simulink model "FlutterSuppressionSystem"  (R2022b)
settings: Solver=ode45  StartTime=0  StopTime=15.01  FixedStep=ts  MaxStep=0.003  RelTol=1e-3  EnableMultiTasking=on
model workspace (MAT data in the model file):
  ts = 0.001
undefined symbols (not defined in the file or in its folder): Hecate_Alt, Hecate_Mach, X, Y, Z
libraries: nesl_utility x14, sm_lib x11, simulink x3, aerolibprivatev1p5 x1, aerolibasang x1
settings Model: Creator=The MathWorks, Inc.  LastModifiedBy=fedformi_new
settings SolverCC: ConcurrentTasks=on  AlgebraicLoopSolver=TrustRegion  PositivePriorityOrder=on  AutoInsertRateTranBlk=on  InsertRTBMode=Never (minimum delay)
settings DataIOCC: SaveFormat=Array  TimeSaveName=tOut  OutputSaveName=yOut  SignalLoggingName=sigsOut
settings OptimizationCC: BlockReduction=off  OptimizeBlockIOStorage=off  BufferReuse=off  GlobalBufferReuse=off  ExpressionFolding=off  ExpressionDepthLimit=2147483647  LocalBlockOutputs=off  InitFltsAndDblsToZero=on  OptimizeDataStoreBuffers=off  BusAssignmentInplaceUpdate=off
settings DebuggingCC: AlgebraicLoopMsg=none  SaveWithParameterizedLinksMsg=none  UnderspecifiedInitializationDetection=Classic  MergeDetectMultiDrivingBlocksExec=none  SignalResolutionControl=TryResolveAllWithWarning  FcnCallInpInsideContextMsg=warning  StateNameClashWarn=warning  SFUnexpectedBacktrackingDiag=warning  SFNoUnconditionalDefaultTransitionDiag=warning  SFExecutionAtInitializationDiag=none  SFMachineParentedDataDiag=warning  ArithmeticOperatorsInVariantConditions=warning
settings ModelReferenceCC: EnableRefExpFcnMdlSchedulingChecks=on  PropagateSignalLabelsOutOfModel=off
settings SFSimCC: SimUseLocalCustomCode=off  SimParseCustomCode=off  CustomCodeUndefinedFunction=UseInterfaceOnly
settings RTWCC: RTWUseLocalCustomCode=off  BuildConfiguration=Faster Runs  DLArmComputeVersion=19.05
settings CodeAppCC: StateflowObjectComments=on
settings ConfigComp: CovMetricSettings=dw  CovSaveCumulativeToWorkspaceVar=on  CovSaveSingleToWorkspaceVar=on  CovExternalEMLEnable=off  CovSFcnEnable=off
settings SimscapeCC: SimscapeNormalizeSystem=off
settings ConfigurationSet: Description=SimMechanics 2G
settings ExplorerConfigSet: SimMechanicsOpenEditorOnUpdate=off

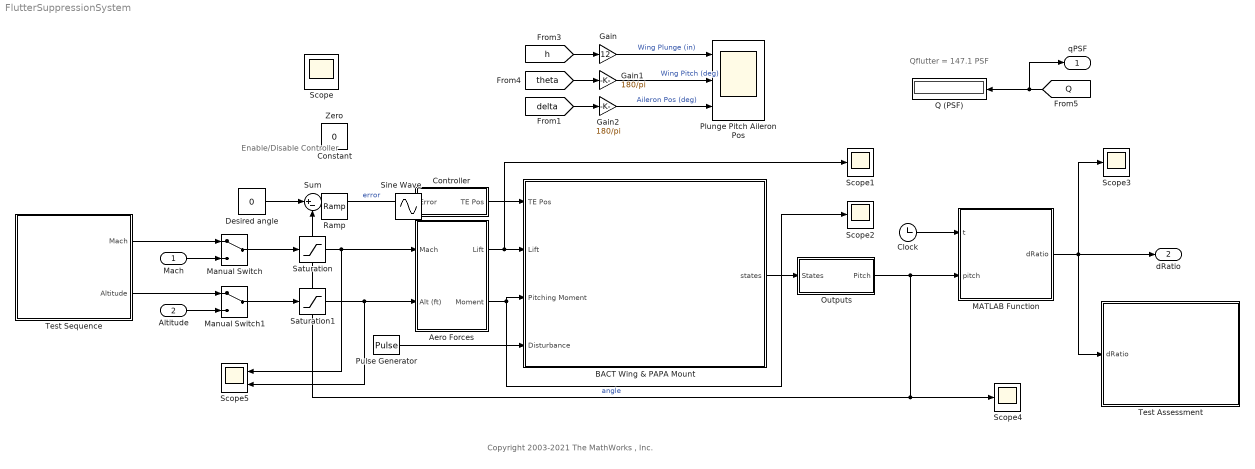
== system FlutterSuppressionSystem ==
  note: Copyright 2003-2021 The MathWorks , Inc.
  note: Enable/Disable Controller
  note: Qflutter = 147.1 PSF
  Mach : Inport
  Altitude : Inport  Port=2
  Aero Forces : Subsystem
  BACT Wing & PAPA Mount : Subsystem  mask{m=6.08, iyy=2.8, Kp=2686.0, zetaP=.0014*2*6.08*21.01, Kt=3000.0, zetaT=.001*2*2.8*32.71, xcg=-.175/100*1.33}
      mask prompts: m "Mass (slug)"; iyy "Inertia (slug*ft^2)"; Kp "PAPA Plunge Stiffness (lb/ft)"; zetaP "PAPA Plunge Damping"; Kt "PAPA Pitch Stiffness (ft-lb)"; zetaT "PAPA Pitch Damping"; xcg "CG Distance from Elastic Axis (+aft)"
      mask Display:
      | image('BACTwing.jpg')
      | port_label('input',1,'TE Position (deg)')
      | port_label('input',2,'Lift')
      | port_label('input',3,'Pitching Moment')
      | port_label('input',4,'Initial Disturbance')
      | port_label('output',1,'States')
  Clock : Clock
  Controller : Subsystem
  Desired angle : Constant  Value=0
  Gain : Gain  Gain=12
  Gain1 : Gain  Gain=180/pi
  Gain2 : Gain  Gain=180/pi
  MATLAB Function : MATLAB Function  TreatAsAtomicUnit=on
  Manual Switch : ManualSwitch
  Manual Switch1 : ManualSwitch
  Outputs : Subsystem
  Plunge Pitch Aileron Pos : Scope  NumInputPorts=3
  Pulse Generator : DiscretePulseGenerator  PulseType=Time based  Amplitude=-10+3*rand  Period=30  PulseWidth=0.05  PhaseDelay=2+3*rand
  Q (PSF) : Display
  Saturation : Saturate  UpperLimit=1  LowerLimit=0.1
  Saturation1 : Saturate  UpperLimit=51000  LowerLimit=1000
  Scope{,1..4} (5 alike) : Scope
  Scope5 : Scope  NumInputPorts=2
  Sum : Sum  Inputs=|+-
  Test Assessment : Test Sequence  TreatAsAtomicUnit=on
  Test Sequence : Test Sequence  TreatAsAtomicUnit=on
  qPSF : Outport  VectorParamsAs1DForOutWhenUnconnected=off
  dRatio : Outport  Port=2
  Constant : Constant  IOType=siggen  Value=-1
  Ramp : simulink/Sources/Ramp  IOType=siggen  slope=1  start=0  InitialOutput=0
  Sine Wave : Sin  IOType=siggen  Amplitude=10  Frequency=5  Phase=pi/2  SampleTime=0
  Zero : Constant  IOType=siggen  Value=0
  wires:
  Manual Switch1/1 -> Saturation1/1
  Manual Switch/1 -> Saturation/1
  BACT Wing & PAPA Mount/1(states) -> Outputs/1(States)
  [Q] -> Q (PSF)/1, qPSF/1
  [h] -> Gain/1
  [theta] -> Gain1/1
  Gain/1 -> Plunge Pitch Aileron Pos/1  "Wing Plunge (in)"
  Gain1/1 -> Plunge Pitch Aileron Pos/2  "Wing Pitch (deg)"
  Sum/1 -> Controller/1(Error)  "error"
  Outputs/1(Pitch) -> MATLAB Function/2(pitch), Sum/2, Scope4/1  "angle"
  Controller/1(TE Pos) -> BACT Wing & PAPA Mount/1(TE Pos)
  [delta] -> Gain2/1
  Gain2/1 -> Plunge Pitch Aileron Pos/3  "Aileron Pos (deg)"
  Desired angle/1 -> Sum/1
  Pulse Generator/1 -> BACT Wing & PAPA Mount/4(Disturbance)
  Aero Forces/1(Lift) -> Scope1/1, BACT Wing & PAPA Mount/2(Lift)
  Aero Forces/2(Moment) -> BACT Wing & PAPA Mount/3(Pitching Moment), Scope2/1
  Clock/1 -> MATLAB Function/1(t)
  Test Sequence/1(Mach) -> Manual Switch/1
  Mach/1 -> Manual Switch/2
  Test Sequence/2(Altitude) -> Manual Switch1/1
  Altitude/1 -> Manual Switch1/2
  MATLAB Function/1(dRatio) -> Scope3/1, dRatio/1, Test Assessment/1(dRatio)
  Saturation/1 -> Scope5/1, Aero Forces/1(Mach)
  Saturation1/1 -> Scope5/2, Aero Forces/2(Alt (ft))

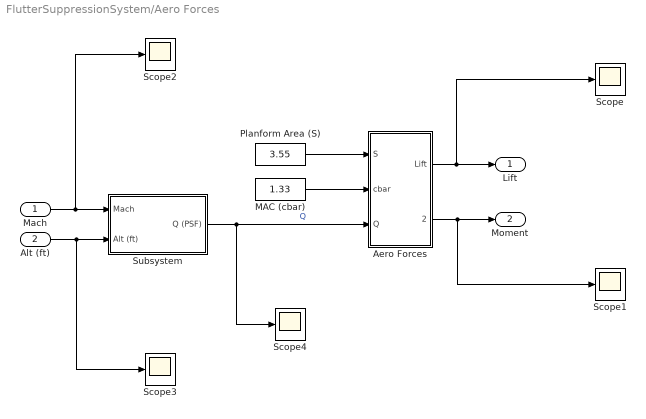
== system FlutterSuppressionSystem/Aero Forces ==
  Mach : Inport
  Alt (ft) : Inport  Port=2
  Aero Forces : Subsystem
  MAC (cbar) : Constant  Value=1.33
  Planform Area (S) : Constant  Value=3.55
  Scope{,1..4} (5 alike) : Scope
  Subsystem : Subsystem
  Lift : Outport  VectorParamsAs1DForOutWhenUnconnected=off
  Moment : Outport  Port=2  VectorParamsAs1DForOutWhenUnconnected=off
  wires:
  MAC (cbar)/1 -> Aero Forces/2(cbar)
  Planform Area (S)/1 -> Aero Forces/1(S)
  Subsystem/1(Q (PSF)) -> Scope4/1, Aero Forces/3(Q)  "Q"
  Aero Forces/1(Lift) -> Scope/1, Lift/1
  Mach/1 -> Scope2/1, Subsystem/1(Mach)
  Aero Forces/2(Moment) -> Scope1/1, Moment/1
  Alt (ft)/1 -> Scope3/1, Subsystem/2(Alt (ft))

== system FlutterSuppressionSystem/BACT Wing & PAPA Mount ==
  TE Pos : Inport
  Lift : Inport  Port=2
  Pitching Moment : Inport  Port=3
  Disturbance : Inport  Port=4
  Bus Creator : BusCreator  Inputs=6
  Mux1 : Mux  Inputs=6
  Sum : Sum  Inputs=++|
  Trailing Edge : Subsystem
  Wing/PAPA Mount : Subsystem
  states : Outport  VectorParamsAs1DForOutWhenUnconnected=off
  wires:
  Bus Creator/1 -> states/1
  Mux1/1 -> Wing/PAPA Mount/1(Aerodynamic Forces)
  Lift/1 -> Mux1/5
  Pitching Moment/1 -> Sum/2
  Sum/1 -> Mux1/3
  Wing/PAPA Mount/1(h) -> Bus Creator/1
  Wing/PAPA Mount/2(hDot) -> Bus Creator/2
  Wing/PAPA Mount/3(theta) -> Bus Creator/3
  Wing/PAPA Mount/4(thetaDot) -> Bus Creator/4
  Trailing Edge/1(delta) -> Bus Creator/5
  Trailing Edge/2(deltaDot) -> Bus Creator/6
  TE Pos/1 -> Trailing Edge/1(TE Pos)
  Disturbance/1 -> Sum/1
  connections:
  Trailing Edge/LConn1 -- Wing/PAPA Mount/RConn1

== system FlutterSuppressionSystem/Controller ==
  Error : Inport
  Constant : Constant
  Enabled Subsystem : Subsystem  TreatAsAtomicUnit=on
  Physical Constraints : Subsystem  mask(Physical Constraint Block){satLimit=15, rateLimit=15/.05*2}
      mask prompts: satLimit "Maximum Deflection (+/- n deg)"; rateLimit "Maximum Deflection Rate (+/- n deg/sec)"
      mask help:
      | In place of an actual actuator model, this block enforces the following constraints:
      | 1 - Maximum/Minimum deflection angle in degrees.
      | 2 - Maximum deflection rate in degrees/sec.
  on/off : Gain  Gain=1.0
  TE Pos : Outport  VectorParamsAs1DForOutWhenUnconnected=off
  wires:
  Enabled Subsystem/1(teCMD) -> Physical Constraints/1(command)  "TE command"
  Error/1 -> Enabled Subsystem/1(error)
  Physical Constraints/1(actual) -> TE Pos/1
  on/off/1 -> Enabled Subsystem/Enable
  Constant/1 -> on/off/1

== system FlutterSuppressionSystem/Outputs ==
  States : Inport
  Bus Selector : BusSelector  OutputSignals=h,hDot,theta,thetaDot,delta,deltaDot
  Memory : Memory
  Pitch : Outport  VectorParamsAs1DForOutWhenUnconnected=off
  tag scope: delta=global, deltaDot=global, h=global, hDot=global, theta=global, thetaDot=global
  wires:
  Bus Selector/1 -> [h]  "<h>"
  Bus Selector/2 -> [hDot]  "<hDot>"
  Bus Selector/3 -> [theta], Memory/1  "<theta>"
  Bus Selector/4 -> [thetaDot]  "<thetaDot>"
  Bus Selector/5 -> [delta]  "<delta>"
  Bus Selector/6 -> [deltaDot]  "<deltaDot>"
  States/1 -> Bus Selector/1
  Memory/1 -> Pitch/1

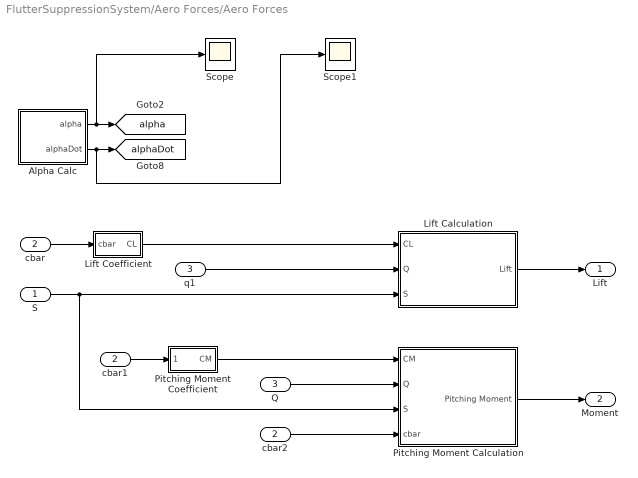
== system FlutterSuppressionSystem/Aero Forces/Aero Forces ==
  S : Inport
  cbar : Inport  Port=2
  Q : Inport  Port=3
  Alpha Calc : Subsystem
  Lift Coefficient : Subsystem
  Lift Calculation : Subsystem
  Pitching Moment Coefficient : Subsystem
  Pitching Moment Calculation : Subsystem
  Scope : Scope
  Scope1 : Scope
  cbar1 : InportShadow  Port=2
  cbar2 : InportShadow  Port=2
  q1 : InportShadow  Port=3
  Lift : Outport  VectorParamsAs1DForOutWhenUnconnected=off
  Moment : Outport  Port=2  VectorParamsAs1DForOutWhenUnconnected=off
  tag scope: alpha=global, alphaDot=global
  wires:
  Lift Coefficient/1(CL) -> Lift Calculation/1(CL)
  q1/1 -> Lift Calculation/2(Q)
  Pitching Moment Coefficient/1(CM) -> Pitching Moment Calculation/1(CM)
  S/1 -> Pitching Moment Calculation/3(S), Lift Calculation/3(S)
  Lift Calculation/1(Lift) -> Lift/1
  Pitching Moment Calculation/1(Pitching Moment) -> Moment/1
  Q/1 -> Pitching Moment Calculation/2(Q)
  cbar/1 -> Lift Coefficient/1(cbar)
  cbar1/1 -> Pitching Moment Coefficient/1(cbar)
  cbar2/1 -> Pitching Moment Calculation/4(cbar)
  Alpha Calc/2(alphaDot) -> Scope1/1, [alphaDot]
  Alpha Calc/1(alpha) -> Scope/1, [alpha]

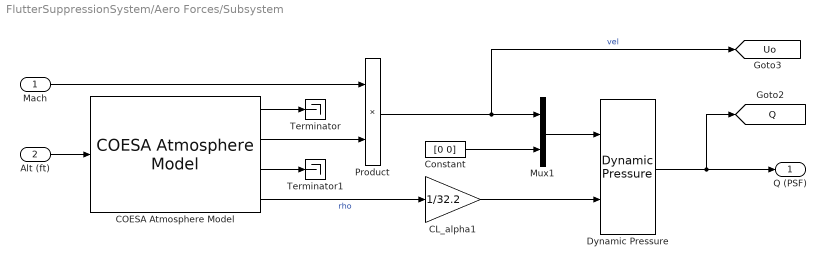
== system FlutterSuppressionSystem/Aero Forces/Subsystem ==
  Mach : Inport
  Alt (ft) : Inport  Port=2
  CL_alpha1 : Gain  Gain=1/32.2  SaturateOnIntegerOverflow=on  OutDataTypeStr=Inherit: Same as input  ParamDataTypeStr=Inherit: Same as input
  COESA Atmosphere Model : aerolibprivatev1p5/COESA Atmosphere Model  units=English
  Constant : Constant  Value=[0 0]
  Dynamic Pressure : aerolibasang/Dynamic Pressure
  Mux1 : Mux  Inputs=2
  Product : Product  SaturateOnIntegerOverflow=on  OutDataTypeStr=Inherit: Same as first input
  Terminator : Terminator
  Terminator1 : Terminator
  Q (PSF) : Outport  VectorParamsAs1DForOutWhenUnconnected=off
  tag scope: Q=global, Uo=global
  wires:
  COESA Atmosphere Model/1 -> Terminator/1
  COESA Atmosphere Model/3 -> Terminator1/1
  COESA Atmosphere Model/2 -> Product/2
  COESA Atmosphere Model/4 -> CL_alpha1/1  "rho"
  Product/1 -> [Uo], Mux1/1  "vel"
  Alt (ft)/1 -> COESA Atmosphere Model/1
  Constant/1 -> Mux1/2
  Mach/1 -> Product/1
  Mux1/1 -> Dynamic Pressure/1
  CL_alpha1/1 -> Dynamic Pressure/2
  Dynamic Pressure/1 -> [Q], Q (PSF)/1

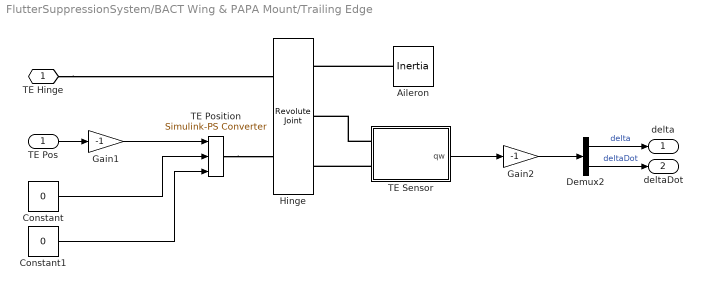
== system FlutterSuppressionSystem/BACT Wing & PAPA Mount/Trailing Edge ==
  TE Pos : Inport
  Aileron : sm_lib/Body Elements/Inertia  InertiaType=Custom  Mass=(1e-9)*14.5939  MassUnits=kg  CenterOfMass=[-8 0 0]  CenterOfMassUnits=in  MomentsOfInertia=([1 1 1]*1e-9)*1.35581795  MomentsOfInertiaUnits=kg*m^2  ProductsOfInertia=[0 0 0]  ProductsOfInertiaUnits=kg*m^2  GraphicType=Marker  MarkerShape=Inertia  MarkerSize=20  GraphicVisPropType=SimpleVisualProperties  GraphicDiffuseColor=[0.5 0.5 0.5]  GraphicSpecularColor=[0.5 0.5 0.5 1.0]  GraphicAmbientColor=[0.15 0.15 0.15 1.0]  GraphicEmissiveColor=[0.0 0.0 0.0 1.0]  GraphicShininess=75  GraphicOpacity=1.0
  Constant : Constant  Value=0
  Constant1 : Constant  Value=0
  Demux2 : Demux  Outputs=2
  Gain1 : Gain  Gain=-1
  Gain2 : Gain  Gain=-1
  Hinge : sm_lib/Joints/Revolute Joint  JointMode=Normal  SenseConstraintForce=off  SenseConstraintForceX=off  SenseConstraintForceY=off  SenseConstraintForceZ=off  SenseConstraintTorque=off  SenseConstraintTorqueX=off  SenseConstraintTorqueY=off  SenseConstraintTorqueZ=off  SenseTotalForce=off  SenseTotalForceX=off  SenseTotalForceY=off  SenseTotalForceZ=off  SenseTotalTorque=off  SenseTotalTorqueX=off  SenseTotalTorqueY=off  SenseTotalTorqueZ=off  CompositeWrenchDir=FollowerOnBase  CompositeWrenchFrame=BaseFrame  EquilibriumPosition=0  EquilibriumPositionUnits=deg  SpringStiffness=0  SpringStiffnessUnits=N*m/deg  DampingCoefficient=0  DampingCoefficientUnits=N*m/(deg/s)  TorqueActuationMode=ComputedTorque  MotionActuationMode=InputMotion  SensePosition=on  SenseVelocity=on  SenseAcceleration=off  SenseTorqueForce=off  SenseLowerLimitTorqueForce=off  SenseUpperLimitTorqueForce=off  LowerLimitSpecify=off  LowerLimitBound=-90  LowerLimitBoundUnits=deg  LowerLimitStiffness=1e4  LowerLimitStiffnessUnits=N*m/deg  LowerLimitDamping=10  LowerLimitDampingUnits=N*m/(deg/s)  LowerLimitTransitionRegionWidth=0.1  LowerLimitTransitionRegionWidthUnits=deg  UpperLimitSpecify=off  UpperLimitBound=90  UpperLimitBoundUnits=deg  UpperLimitStiffness=1e4  UpperLimitStiffnessUnits=N*m/deg  UpperLimitDamping=10  UpperLimitDampingUnits=N*m/(deg/s)  UpperLimitTransitionRegionWidth=0.1  UpperLimitTransitionRegionWidthUnits=deg  PositionTargetSpecify=off  PositionTargetPriority=High  PositionTargetValue=0  PositionTargetValueUnits=deg  VelocityTargetSpecify=off  VelocityTargetPriority=High  VelocityTargetValue=0  VelocityTargetValueUnits=deg/s
  TE Position : nesl_utility/Simulink-PS Converter  PhysicalDomain=network_engine_domain  SubClassName=ps_input  LeftPortType=input  RightPortType=output  PseudoPeriodic=off  Frequencies=[]  NoiseDistribution=none  NoiseParameters=[]  Unit=deg  AffineConversion=off  FilteringAndDerivatives=provide  SimscapeFilterOrder=2  InputFilterTimeConstant=0.001  UdotUserProvided=2
  TE Sensor : Subsystem
  TE Hinge : PMIOPort  Side=Left
  delta : Outport  VectorParamsAs1DForOutWhenUnconnected=off
  deltaDot : Outport  Port=2  VectorParamsAs1DForOutWhenUnconnected=off
  wires:
  Gain2/1 -> Demux2/1
  TE Pos/1 -> Gain1/1
  Demux2/1 -> delta/1  "delta"
  Demux2/2 -> deltaDot/1  "deltaDot"
  Gain1/1 -> TE Position/1
  TE Sensor/1(qw) -> Gain2/1
  Constant/1 -> TE Position/2
  Constant1/1 -> TE Position/3
  connections:
  TE Position/RConn1 -- Hinge/LConn2
  Aileron/RConn1 -- Hinge/RConn1
  TE Sensor/LConn1 -- Hinge/RConn2
  TE Sensor/LConn2 -- Hinge/RConn3
  TE Hinge/RConn1 -- Hinge/LConn1

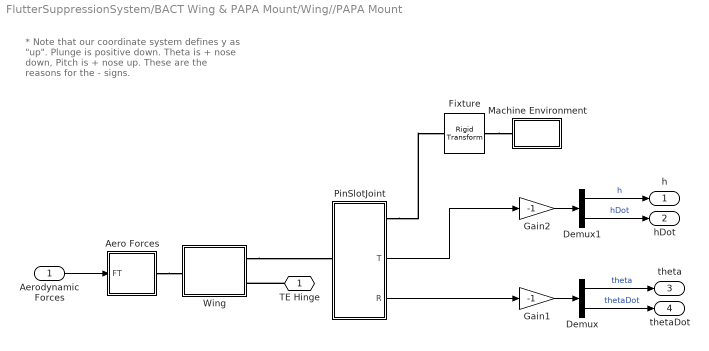
== system FlutterSuppressionSystem/BACT Wing & PAPA Mount/Wing//PAPA Mount ==
  note: * Note that our coordinate system
      | defines y as "up".  Plunge is positive down.
      | Theta is + nose down, Pitch is + nose up.
      | These are the reasons for the - signs.
  Aerodynamic Forces : Inport
  Aero Forces : Subsystem
  Demux : Demux  Outputs=2
  Demux1 : Demux  Outputs=2
  Fixture : sm_lib/Frames and Transforms/Rigid Transform  TranslationMethod=Cartesian  TranslationStandardOffset=0  TranslationLengthUnit=in  TranslationStandardAxis=+Z  TranslationCartesianOffset=[4 0 0]  TranslationROffset=0  TranslationROffsetUnits=m  TranslationZOffset=0  TranslationZOffsetUnits=m  TranslationThetaOffset=0  TranslationThetaOffsetUnits=deg  RotationMethod=None  RotationAngleUnits=deg  RotationStandardAxis=+Z  RotationAngle=0.0  RotationArbitraryAxis=[0 0 1]  FollAlignAxisA=+X  BaseAlignAxisA=+Y  FollAlignAxisB=+Y  BaseAlignAxisB=+Z  RotationSequenceAxes=FollowerAxes  RotationSequence=XYX  RotationSequenceAngles=[0 0 0]  RotationSequenceAnglesUnits=deg  RotationMatrix=[1 0 0; 0 1 0; 0 0 1]  Quaternion=[1 0 0 0]
  Gain1 : Gain  Gain=-1
  Gain2 : Gain  Gain=-1
  Machine Environment : Subsystem
  PinSlotJoint : Subsystem
      settings: PortSchema="{\"entries\":[{\"content\":{\"sides\":[{\"content\":{\"connectorIds\":[\"LConn1\",\"Out1\",\"Out2\"]},\"type\":\"ConnectorPlacement.EquallySpacedRectSide\",\"uuid\":\"cdb19b1c-c324-4790-bce0-6ea35c5c238f\"},{\"content\":{\"connectorIds\":[\"RConn1\"],\"side\":\"RIGHT\"},\"type\":\"ConnectorPlacement.EquallySpacedRectSide\",\"uuid\":\"403fc385-ba39-4b7a-a6e6-6154bbf75764\"},{\"content\":{\"connectorIds\":[],\"side\":\"TOP\"},\"type\":\"ConnectorPlacement.EquallySpacedRectSide\",\"uuid\":\"fec16613-0661-475b-a896-54521c2e84d5\"}]},\"type\":\"ConnectorPlacement.EquallySpacedConnector\",\"uuid\":\"b146dd63-fc25-4a76-acd3-1d9d241f42f8\"}],\"packageUris\":[\"http://schema.mathworks.com/mf0/Connector/19700101\"],\"version\":\"1.0\"}"
  Wing : Subsystem
  TE Hinge : PMIOPort  Side=Right
  h : Outport  VectorParamsAs1DForOutWhenUnconnected=off
  hDot : Outport  Port=2  VectorParamsAs1DForOutWhenUnconnected=off
  theta : Outport  Port=3  VectorParamsAs1DForOutWhenUnconnected=off
  thetaDot : Outport  Port=4  VectorParamsAs1DForOutWhenUnconnected=off
  wires:
  PinSlotJoint/2(R) -> Gain1/1
  PinSlotJoint/1(T) -> Gain2/1
  Demux1/1 -> h/1  "h"
  Demux1/2 -> hDot/1  "hDot"
  Demux/1 -> theta/1  "theta"
  Demux/2 -> thetaDot/1  "thetaDot"
  Gain1/1 -> Demux/1
  Gain2/1 -> Demux1/1
  Aerodynamic Forces/1 -> Aero Forces/1(FT)
  connections:
  Fixture/LConn1 -- Machine Environment/LConn1
  PinSlotJoint/LConn1 -- Fixture/RConn1
  Wing/RConn1 -- PinSlotJoint/RConn1
  Aero Forces/RConn1 -- Wing/LConn1
  TE Hinge/RConn1 -- Wing/RConn2

== system FlutterSuppressionSystem/Controller/Enabled Subsystem ==
  error : Inport
  Enable : EnablePort  StatesWhenEnabling=reset
  Controller : TransferFcn  Numerator=[-10393.7989539677 -80183.6874752132 -565082.359817244]  Denominator=[1 100 0]
  teCMD : Outport  VectorParamsAs1DForOutWhenUnconnected=off
  wires:
  error/1 -> Controller/1
  Controller/1 -> teCMD/1

== system FlutterSuppressionSystem/Controller/Physical Constraints ==
  command : Inport
  Rate Limiter : RateLimiter  RisingSlewLimit=rateLimit  FallingSlewLimit=-rateLimit  SampleTimeMode=inherited
  Saturation : Saturate  UpperLimit=satLimit  LowerLimit=-satLimit
  actual : Outport  VectorParamsAs1DForOutWhenUnconnected=off
  wires:
  Saturation/1 -> Rate Limiter/1
  Rate Limiter/1 -> actual/1
  command/1 -> Saturation/1

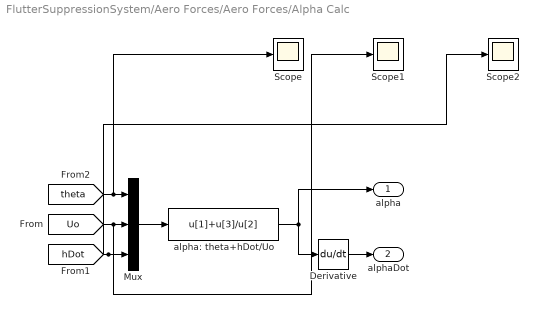
== system FlutterSuppressionSystem/Aero Forces/Aero Forces/Alpha Calc ==
  Derivative : Derivative
  Mux : Mux  Inputs=3
  Scope : Scope
  Scope1 : Scope
  Scope2 : Scope
  alpha: theta+hDot/Uo : Fcn  Expr=u[1]+u[3]/u[2]
  alpha : Outport  VectorParamsAs1DForOutWhenUnconnected=off
  alphaDot : Outport  Port=2  VectorParamsAs1DForOutWhenUnconnected=off
  wires:
  Mux/1 -> alpha: theta+hDot/Uo/1
  alpha: theta+hDot/Uo/1 -> Derivative/1, alpha/1
  [theta] -> Scope/1, Mux/1
  [Uo] -> Scope1/1, Mux/2
  Derivative/1 -> alphaDot/1
  [hDot] -> Mux/3, Scope2/1

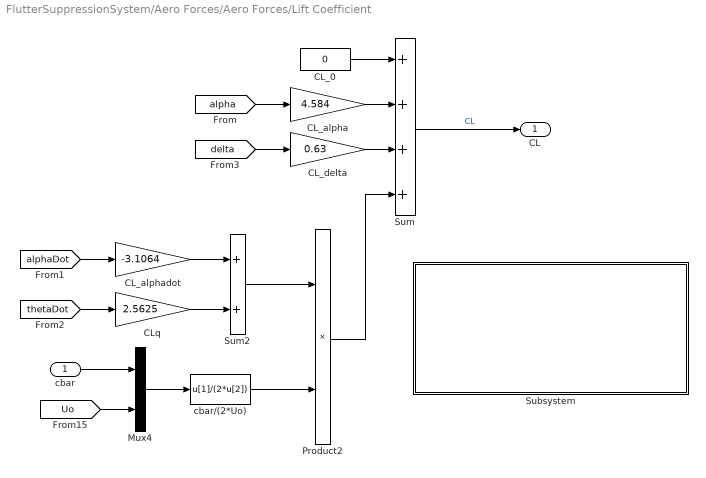
== system FlutterSuppressionSystem/Aero Forces/Aero Forces/Lift Coefficient ==
  cbar : Inport
  CL_0 : Constant  Value=0
  CL_alpha : Gain  Gain=4.584  SaturateOnIntegerOverflow=on  OutDataTypeStr=Inherit: Same as input  ParamDataTypeStr=Inherit: Same as input
  CL_alphadot : Gain  Gain=-3.1064  SaturateOnIntegerOverflow=on  OutDataTypeStr=Inherit: Same as input  ParamDataTypeStr=Inherit: Same as input
  CL_delta : Gain  Gain=0.63  SaturateOnIntegerOverflow=on  OutDataTypeStr=Inherit: Same as input  ParamDataTypeStr=Inherit: Same as input
  CLq : Gain  Gain=2.5625  SaturateOnIntegerOverflow=on  OutDataTypeStr=Inherit: Same as input  ParamDataTypeStr=Inherit: Same as input
  Mux4 : Mux  Inputs=2
  Product2 : Product  SaturateOnIntegerOverflow=on  OutDataTypeStr=Inherit: Same as first input
  Subsystem : Subsystem
      mask Display: image('LiftEquation.jpg')
  Sum : Sum  Inputs=++++  SaturateOnIntegerOverflow=on
  Sum2 : Sum  SaturateOnIntegerOverflow=on
  cbar/(2*Uo) : Fcn  Expr=u[1]/(2*u[2])
  CL : Outport  VectorParamsAs1DForOutWhenUnconnected=off
  wires:
  [alpha] -> CL_alpha/1
  CL_0/1 -> Sum/1
  CL_alpha/1 -> Sum/2
  [alphaDot] -> CL_alphadot/1
  [thetaDot] -> CLq/1
  CL_alphadot/1 -> Sum2/1
  CLq/1 -> Sum2/2
  Sum2/1 -> Product2/1
  cbar/1 -> Mux4/1
  [Uo] -> Mux4/2
  Mux4/1 -> cbar/(2*Uo)/1
  cbar/(2*Uo)/1 -> Product2/2
  Sum/1 -> CL/1  "CL"
  Product2/1 -> Sum/4
  [delta] -> CL_delta/1
  CL_delta/1 -> Sum/3

== system FlutterSuppressionSystem/Aero Forces/Aero Forces/Lift Calculation ==
  CL : Inport
  Q : Inport  Port=2
  S : Inport  Port=3
  Product : Product  Inputs=3  SaturateOnIntegerOverflow=on  OutDataTypeStr=Inherit: Same as first input
  Lift : Outport  VectorParamsAs1DForOutWhenUnconnected=off
  wires:
  CL/1 -> Product/1
  Q/1 -> Product/2
  S/1 -> Product/3
  Product/1 -> Lift/1

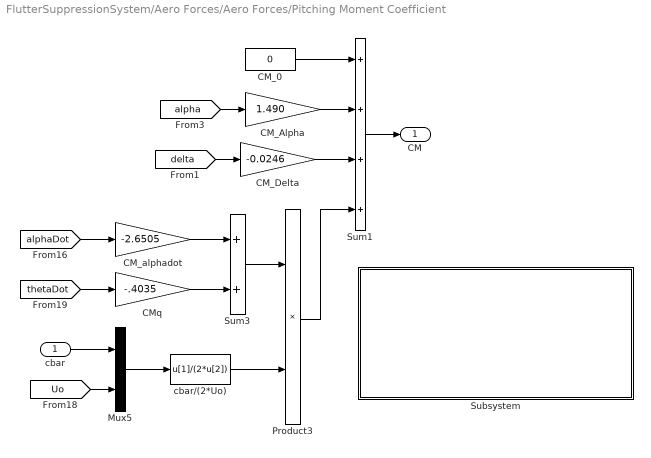
== system FlutterSuppressionSystem/Aero Forces/Aero Forces/Pitching Moment Coefficient ==
  cbar : Inport
  CM_0 : Constant  Value=0
  CM_Alpha : Gain  Gain=1.490  SaturateOnIntegerOverflow=on  OutDataTypeStr=Inherit: Same as input  ParamDataTypeStr=Inherit: Same as input
  CM_Delta : Gain  Gain=-0.0246  SaturateOnIntegerOverflow=on  OutDataTypeStr=Inherit: Same as input  ParamDataTypeStr=Inherit: Same as input
  CM_alphadot : Gain  Gain=-2.6505  SaturateOnIntegerOverflow=on  OutDataTypeStr=Inherit: Same as input  ParamDataTypeStr=Inherit: Same as input
  CMq : Gain  Gain=-.4035  SaturateOnIntegerOverflow=on  OutDataTypeStr=Inherit: Same as input  ParamDataTypeStr=Inherit: Same as input
  Mux5 : Mux  Inputs=2
  Product3 : Product  SaturateOnIntegerOverflow=on  OutDataTypeStr=Inherit: Same as first input
  Subsystem : Subsystem
      mask Display: image('MomentEquation.jpg')
  Sum1 : Sum  Inputs=++++  SaturateOnIntegerOverflow=on
  Sum3 : Sum  SaturateOnIntegerOverflow=on
  cbar/(2*Uo) : Fcn  Expr=u[1]/(2*u[2])
  CM : Outport  VectorParamsAs1DForOutWhenUnconnected=off
  wires:
  [alpha] -> CM_Alpha/1
  CM_Alpha/1 -> Sum1/2
  CM_0/1 -> Sum1/1
  [alphaDot] -> CM_alphadot/1
  [thetaDot] -> CMq/1
  CM_alphadot/1 -> Sum3/1
  CMq/1 -> Sum3/2
  Sum3/1 -> Product3/1
  cbar/1 -> Mux5/1
  [Uo] -> Mux5/2
  Mux5/1 -> cbar/(2*Uo)/1
  cbar/(2*Uo)/1 -> Product3/2
  Sum1/1 -> CM/1
  Product3/1 -> Sum1/4
  [delta] -> CM_Delta/1
  CM_Delta/1 -> Sum1/3

== system FlutterSuppressionSystem/Aero Forces/Aero Forces/Pitching Moment Calculation ==
  CM : Inport
  Q : Inport  Port=2
  S : Inport  Port=3
  cbar : Inport  Port=4
  CL_alpha2 : Gain  Gain=-1  SaturateOnIntegerOverflow=on  OutDataTypeStr=Inherit: Same as input  ParamDataTypeStr=Inherit: Same as input
  Product1 : Product  Inputs=4  SaturateOnIntegerOverflow=on  OutDataTypeStr=Inherit: Same as first input
  Pitching Moment : Outport  VectorParamsAs1DForOutWhenUnconnected=off
  wires:
  Product1/1 -> CL_alpha2/1
  CL_alpha2/1 -> Pitching Moment/1
  CM/1 -> Product1/1
  Q/1 -> Product1/2
  S/1 -> Product1/3
  cbar/1 -> Product1/4

== system FlutterSuppressionSystem/BACT Wing & PAPA Mount/Trailing Edge/TE Sensor ==
  Mux : Mux  Inputs=2
  PS-Simulink Converter : nesl_utility/PS-Simulink Converter  PhysicalDomain=network_engine_domain  SubClassName=ps_output  LeftPortType=input  RightPortType=output  PseudoPeriodic=off  Frequencies=[]  VectorFormat=1-D array  Unit=rad  AffineConversion=off
  PS-Simulink Converter1 : nesl_utility/PS-Simulink Converter  PhysicalDomain=network_engine_domain  SubClassName=ps_output  LeftPortType=input  RightPortType=output  PseudoPeriodic=off  Frequencies=[]  VectorFormat=1-D array  Unit=rad/s  AffineConversion=off
  q : PMIOPort  Side=Left
  w : PMIOPort  Port=2  Side=Left
  qw : Outport
  wires:
  PS-Simulink Converter/1 -> Mux/1
  PS-Simulink Converter1/1 -> Mux/2
  Mux/1 -> qw/1
  connections:
  PS-Simulink Converter/LConn1 -- q/RConn1
  PS-Simulink Converter1/LConn1 -- w/RConn1

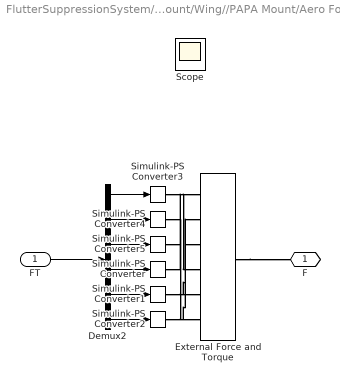
== system FlutterSuppressionSystem/BACT Wing & PAPA Mount/Wing//PAPA Mount/Aero Forces ==
  FT : Inport
  Demux2 : Demux  Outputs=6
  External Force and Torque : sm_lib/Forces and Torques/External Force and Torque  ForceResolutionFrame=World  EnableForceX=on  EnableForceY=on  EnableForceZ=on  EnableForce=off  TorqueResolutionFrame=World  EnableTorqueX=on  EnableTorqueY=on  EnableTorqueZ=on  EnableTorque=off
  Scope : Scope
  Simulink-PS Converter : nesl_utility/Simulink-PS Converter  PhysicalDomain=network_engine_domain  SubClassName=ps_input  LeftPortType=input  RightPortType=output  PseudoPeriodic=off  Frequencies=[]  NoiseDistribution=none  NoiseParameters=[]  Unit=lbf  AffineConversion=off  FilteringAndDerivatives=provide  SimscapeFilterOrder=1  InputFilterTimeConstant=0.001  UdotUserProvided=0
  Simulink-PS Converter1 : nesl_utility/Simulink-PS Converter  PhysicalDomain=network_engine_domain  SubClassName=ps_input  LeftPortType=input  RightPortType=output  PseudoPeriodic=off  Frequencies=[]  NoiseDistribution=none  NoiseParameters=[]  Unit=lbf  AffineConversion=off  FilteringAndDerivatives=provide  SimscapeFilterOrder=1  InputFilterTimeConstant=0.001  UdotUserProvided=0
  Simulink-PS Converter2 : nesl_utility/Simulink-PS Converter  PhysicalDomain=network_engine_domain  SubClassName=ps_input  LeftPortType=input  RightPortType=output  PseudoPeriodic=off  Frequencies=[]  NoiseDistribution=none  NoiseParameters=[]  Unit=lbf  AffineConversion=off  FilteringAndDerivatives=provide  SimscapeFilterOrder=1  InputFilterTimeConstant=0.001  UdotUserProvided=0
  Simulink-PS Converter3 : nesl_utility/Simulink-PS Converter  PhysicalDomain=network_engine_domain  SubClassName=ps_input  LeftPortType=input  RightPortType=output  PseudoPeriodic=off  Frequencies=[]  NoiseDistribution=none  NoiseParameters=[]  Unit=ft*lbf  AffineConversion=off  FilteringAndDerivatives=provide  SimscapeFilterOrder=1  InputFilterTimeConstant=0.001  UdotUserProvided=0
  Simulink-PS Converter4 : nesl_utility/Simulink-PS Converter  PhysicalDomain=network_engine_domain  SubClassName=ps_input  LeftPortType=input  RightPortType=output  PseudoPeriodic=off  Frequencies=[]  NoiseDistribution=none  NoiseParameters=[]  Unit=ft*lbf  AffineConversion=off  FilteringAndDerivatives=provide  SimscapeFilterOrder=1  InputFilterTimeConstant=0.001  UdotUserProvided=0
  Simulink-PS Converter5 : nesl_utility/Simulink-PS Converter  PhysicalDomain=network_engine_domain  SubClassName=ps_input  LeftPortType=input  RightPortType=output  PseudoPeriodic=off  Frequencies=[]  NoiseDistribution=none  NoiseParameters=[]  Unit=ft*lbf  AffineConversion=off  FilteringAndDerivatives=provide  SimscapeFilterOrder=1  InputFilterTimeConstant=0.001  UdotUserProvided=0
  F : PMIOPort  Side=Right
  wires:
  FT/1 -> Demux2/1
  Demux2/1 -> Simulink-PS Converter3/1
  Demux2/2 -> Simulink-PS Converter4/1
  Demux2/3 -> Simulink-PS Converter5/1
  Demux2/4 -> Simulink-PS Converter/1
  Demux2/5 -> Simulink-PS Converter1/1
  Demux2/6 -> Simulink-PS Converter2/1
  connections:
  External Force and Torque/RConn1 -- F/RConn1
  Simulink-PS Converter3/RConn1 -- External Force and Torque/LConn4
  Simulink-PS Converter4/RConn1 -- External Force and Torque/LConn5
  Simulink-PS Converter5/RConn1 -- External Force and Torque/LConn6
  Simulink-PS Converter/RConn1 -- External Force and Torque/LConn1
  Simulink-PS Converter1/RConn1 -- External Force and Torque/LConn2
  Simulink-PS Converter2/RConn1 -- External Force and Torque/LConn3

== system FlutterSuppressionSystem/BACT Wing & PAPA Mount/Wing//PAPA Mount/Machine Environment ==
  Mechanism Configuration : sm_lib/Utilities/Mechanism Configuration  UniformGravity=None  GravityVector=[0 0 -9.80665]  GravityUnits=m/s^2  LinearizationDelta=0.001  JointModeTransitionNonlinearIterations=2
  Solver Configuration : nesl_utility/Solver Configuration  PhysicalDomain=network_engine_domain  SubClassName=solver  LeftPortType=input  RightPortType=generic  Tones=[]  Harmonics=[]  SimulateNoise=off  Profile=off  UseLocalSampling=off  EnableSwitchedLinearOptims=on  FrequencyDomain=off  UseCCode=off  RelTol=0.001  AbsTol=1e-06  MinStep=1e-09  ToWorkspace=off  RevertToSquareIcSolve=off  NumHomotopyIterations=100  PhasorMode=off  PhasorModeNumHarmonics=1  ConsistencySolver=NEWTON_FTOL  IndexReductionMethod=DerivativeReplacement  DoDC=off  ResidualTolerance=1e-09  ConsistencyTolSource=GLOBAL  ConsistencyAbsTol=0.001  ConsistencyRelTol=0.001  ConsistencyTolFactor=0.001  UseLocalSolver=off  LocalSolverChoice=NE_BACKWARD_EULER_ADVANCER  ResolveIndetEquations=on  FunctionEvalNumThread=1  LocalSolverSampleTime=0.001  DoFixedCost=off  MaxNonlinIter=3  MaxModeIter=2  ComputeImpulses=off  ImpulseIterations=1  LinearAlgebra=auto  LinearAlgebraNumThread=0  EquationFormulation=NE_TIME_EF  DelaysMemoryBudget=1024  AutomaticFiltering=on  FilteringTimeConstant=0.001  PartitionStorageMethod=AS_NEEDED  PartitionMemoryBudget=1024  PartitionMethod=ROBUST
  World Frame : sm_lib/Frames and Transforms/World Frame
  W : PMIOPort  Side=Left
  connections:
  Solver Configuration/RConn1 -- W/RConn1 -- Mechanism Configuration/RConn1 -- World Frame/RConn1

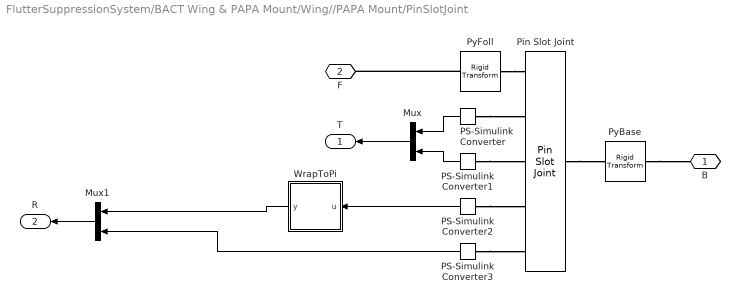
== system FlutterSuppressionSystem/BACT Wing & PAPA Mount/Wing//PAPA Mount/PinSlotJoint ==
  Mux : Mux  Inputs=2
  Mux1 : Mux  Inputs=2
  PS-Simulink Converter : nesl_utility/PS-Simulink Converter  PhysicalDomain=network_engine_domain  SubClassName=ps_output  LeftPortType=input  RightPortType=output  PseudoPeriodic=off  Frequencies=[]  VectorFormat=1-D array  Unit=ft  AffineConversion=off
  PS-Simulink Converter1 : nesl_utility/PS-Simulink Converter  PhysicalDomain=network_engine_domain  SubClassName=ps_output  LeftPortType=input  RightPortType=output  PseudoPeriodic=off  Frequencies=[]  VectorFormat=1-D array  Unit=ft/s  AffineConversion=off
  PS-Simulink Converter2 : nesl_utility/PS-Simulink Converter  PhysicalDomain=network_engine_domain  SubClassName=ps_output  LeftPortType=input  RightPortType=output  PseudoPeriodic=off  Frequencies=[]  VectorFormat=1-D array  Unit=rad  AffineConversion=off
  PS-Simulink Converter3 : nesl_utility/PS-Simulink Converter  PhysicalDomain=network_engine_domain  SubClassName=ps_output  LeftPortType=input  RightPortType=output  PseudoPeriodic=off  Frequencies=[]  VectorFormat=1-D array  Unit=rad/s  AffineConversion=off
  Pin Slot Joint : sm_lib/Joints/Pin Slot Joint  JointMode=Normal  SenseConstraintForce=off  SenseConstraintForceX=off  SenseConstraintForceY=off  SenseConstraintForceZ=off  SenseConstraintTorque=off  SenseConstraintTorqueX=off  SenseConstraintTorqueY=off  SenseConstraintTorqueZ=off  SenseTotalForce=off  SenseTotalForceX=off  SenseTotalForceY=off  SenseTotalForceZ=off  SenseTotalTorque=off  SenseTotalTorqueX=off  SenseTotalTorqueY=off  SenseTotalTorqueZ=off  CompositeWrenchDir=FollowerOnBase  CompositeWrenchFrame=BaseFrame  PxEquilibriumPosition=0  PxEquilibriumPositionUnits=m  PxSpringStiffness=Kp  PxSpringStiffnessUnits=lbf/ft  PxDampingCoefficient=zetaP  PxDampingCoefficientUnits=lbf/(ft/s)  PxTorqueActuationMode=NoTorque  PxMotionActuationMode=ComputedMotion  PxSensePosition=on  PxSenseVelocity=on  PxSenseAcceleration=off  PxSenseTorqueForce=off  PxSenseLowerLimitTorqueForce=off  PxSenseUpperLimitTorqueForce=off  PxLowerLimitSpecify=off  PxLowerLimitBound=-1  PxLowerLimitBoundUnits=m  PxLowerLimitStiffness=1e6  PxLowerLimitStiffnessUnits=N/m  PxLowerLimitDamping=1e3  PxLowerLimitDampingUnits=N/(m/s)  PxLowerLimitTransitionRegionWidth=1e-4  PxLowerLimitTransitionRegionWidthUnits=m  PxUpperLimitSpecify=off  PxUpperLimitBound=1  PxUpperLimitBoundUnits=m  PxUpperLimitStiffness=1e6  PxUpperLimitStiffnessUnits=N/m  PxUpperLimitDamping=1e3  PxUpperLimitDampingUnits=N/(m/s)  PxUpperLimitTransitionRegionWidth=1e-4  PxUpperLimitTransitionRegionWidthUnits=m  PxPositionTargetSpecify=off  PxPositionTargetPriority=High  PxPositionTargetValue=0  PxPositionTargetValueUnits=m  PxVelocityTargetSpecify=off  PxVelocityTargetPriority=High  PxVelocityTargetValue=0  PxVelocityTargetValueUnits=m/s  RzEquilibriumPosition=0  RzEquilibriumPositionUnits=deg  RzSpringStiffness=Kt  RzSpringStiffnessUnits=lbf*ft/rad  RzDampingCoefficient=zetaT  RzDampingCoefficientUnits=lbf*ft/(rad/s)  RzTorqueActuationMode=NoTorque  RzMotionActuationMode=ComputedMotion  RzSensePosition=on  RzSenseVelocity=on  RzSenseAcceleration=off  RzSenseTorqueForce=off  RzSenseLowerLimitTorqueForce=off  RzSenseUpperLimitTorqueForce=off  RzLowerLimitSpecify=off  RzLowerLimitBound=-90  RzLowerLimitBoundUnits=deg  RzLowerLimitStiffness=1e4  RzLowerLimitStiffnessUnits=N*m/deg  RzLowerLimitDamping=10  RzLowerLimitDampingUnits=N*m/(deg/s)  RzLowerLimitTransitionRegionWidth=0.1  RzLowerLimitTransitionRegionWidthUnits=deg  RzUpperLimitSpecify=off  RzUpperLimitBound=90  RzUpperLimitBoundUnits=deg  RzUpperLimitStiffness=1e4  RzUpperLimitStiffnessUnits=N*m/deg  RzUpperLimitDamping=10  RzUpperLimitDampingUnits=N*m/(deg/s)  RzUpperLimitTransitionRegionWidth=0.1  RzUpperLimitTransitionRegionWidthUnits=deg  RzPositionTargetSpecify=off  RzPositionTargetPriority=High  RzPositionTargetValue=0  RzPositionTargetValueUnits=deg  RzVelocityTargetSpecify=off  RzVelocityTargetPriority=High  RzVelocityTargetValue=0  RzVelocityTargetValueUnits=deg/s
  PyBase : sm_lib/Frames and Transforms/Rigid Transform  TranslationMethod=None  TranslationStandardOffset=0  TranslationLengthUnit=m  TranslationStandardAxis=+Z  TranslationCartesianOffset=[0 0 0]  TranslationROffset=0  TranslationROffsetUnits=m  TranslationZOffset=0  TranslationZOffsetUnits=m  TranslationThetaOffset=0  TranslationThetaOffsetUnits=deg  RotationMethod=AlignedAxes  RotationAngleUnits=deg  RotationStandardAxis=+Z  RotationAngle=0.0  RotationArbitraryAxis=[0 0 1]  FollAlignAxisA=+X  BaseAlignAxisA=+Y  FollAlignAxisB=+Z  BaseAlignAxisB=+Z  RotationSequenceAxes=FollowerAxes  RotationSequence=XYX  RotationSequenceAngles=[0 0 0]  RotationSequenceAnglesUnits=deg  RotationMatrix=[1 0 0; 0 1 0; 0 0 1]  Quaternion=[1 0 0 0]
  PyFoll : sm_lib/Frames and Transforms/Rigid Transform  TranslationMethod=None  TranslationStandardOffset=0  TranslationLengthUnit=m  TranslationStandardAxis=+Z  TranslationCartesianOffset=[0 0 0]  TranslationROffset=0  TranslationROffsetUnits=m  TranslationZOffset=0  TranslationZOffsetUnits=m  TranslationThetaOffset=0  TranslationThetaOffsetUnits=deg  RotationMethod=AlignedAxes  RotationAngleUnits=deg  RotationStandardAxis=+Z  RotationAngle=0.0  RotationArbitraryAxis=[0 0 1]  FollAlignAxisA=+Y  BaseAlignAxisA=+X  FollAlignAxisB=+Z  BaseAlignAxisB=+Z  RotationSequenceAxes=FollowerAxes  RotationSequence=XYX  RotationSequenceAngles=[0 0 0]  RotationSequenceAnglesUnits=deg  RotationMatrix=[1 0 0; 0 1 0; 0 0 1]  Quaternion=[1 0 0 0]
  WrapToPi : Subsystem  TreatAsAtomicUnit=on
  B : PMIOPort  Side=Left
  F : PMIOPort  Port=2  Side=Right
  T : Outport
  R : Outport  Port=2
  wires:
  PS-Simulink Converter/1 -> Mux/1
  PS-Simulink Converter1/1 -> Mux/2
  Mux/1 -> T/1
  Mux1/1 -> R/1
  PS-Simulink Converter3/1 -> Mux1/2
  PS-Simulink Converter2/1 -> WrapToPi/1(u)
  WrapToPi/1(y) -> Mux1/1
  connections:
  PyBase/LConn1 -- B/RConn1
  PyFoll/LConn1 -- Pin Slot Joint/RConn1
  PS-Simulink Converter/LConn1 -- Pin Slot Joint/RConn2
  PS-Simulink Converter1/LConn1 -- Pin Slot Joint/RConn3
  PS-Simulink Converter2/LConn1 -- Pin Slot Joint/RConn4
  PS-Simulink Converter3/LConn1 -- Pin Slot Joint/RConn5
  Pin Slot Joint/LConn1 -- PyBase/RConn1
  PyFoll/RConn1 -- F/RConn1

== system FlutterSuppressionSystem/BACT Wing & PAPA Mount/Wing//PAPA Mount/Wing ==
  CS3ToCS2 : sm_lib/Frames and Transforms/Rigid Transform  TranslationMethod=Cartesian  TranslationStandardOffset=0  TranslationLengthUnit=in  TranslationStandardAxis=+Z  TranslationCartesianOffset=[8 0 0]  TranslationROffset=0  TranslationROffsetUnits=m  TranslationZOffset=0  TranslationZOffsetUnits=m  TranslationThetaOffset=0  TranslationThetaOffsetUnits=deg  RotationMethod=None  RotationAngleUnits=deg  RotationStandardAxis=+Z  RotationAngle=0.0  RotationArbitraryAxis=[0 0 1]  FollAlignAxisA=+X  BaseAlignAxisA=+Y  FollAlignAxisB=+Y  BaseAlignAxisB=+Z  RotationSequenceAxes=FollowerAxes  RotationSequence=XYX  RotationSequenceAngles=[0 0 0]  RotationSequenceAnglesUnits=deg  RotationMatrix=[1 0 0; 0 1 0; 0 0 1]  Quaternion=[1 0 0 0]
  Inertia : sm_lib/Body Elements/Inertia  InertiaType=Custom  Mass=m*14.5939  MassUnits=kg  CenterOfMass=[xcg 0 0]  CenterOfMassUnits=in  MomentsOfInertia=[0 0 iyy]*1.35581795  MomentsOfInertiaUnits=kg*m^2  ProductsOfInertia=[0 0 0]  ProductsOfInertiaUnits=kg*m^2  GraphicType=Marker  MarkerShape=Inertia  MarkerSize=20  GraphicVisPropType=SimpleVisualProperties  GraphicDiffuseColor=[0.5 0.5 0.5]  GraphicSpecularColor=[0.5 0.5 0.5 1.0]  GraphicAmbientColor=[0.15 0.15 0.15 1.0]  GraphicEmissiveColor=[0.0 0.0 0.0 1.0]  GraphicShininess=75  GraphicOpacity=1.0
  CS3 : PMIOPort  Side=Right
  CS2 : PMIOPort  Port=2  Side=Right
  CS4 : PMIOPort  Port=3  Side=Left
  connections:
  CS3ToCS2/LConn1 -- Inertia/RConn1 -- CS3/RConn1 -- CS4/RConn1
  CS3ToCS2/RConn1 -- CS2/RConn1

== system FlutterSuppressionSystem/Aero Forces/Aero Forces/Lift Coefficient/Subsystem ==

== system FlutterSuppressionSystem/Aero Forces/Aero Forces/Pitching Moment Coefficient/Subsystem ==

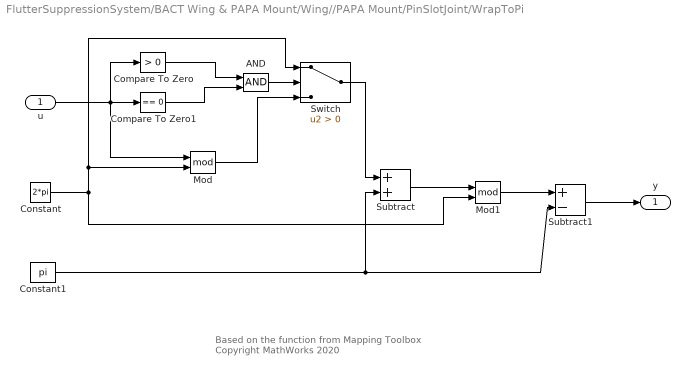
== system FlutterSuppressionSystem/BACT Wing & PAPA Mount/Wing//PAPA Mount/PinSlotJoint/WrapToPi ==
  note: Based on the function from Mapping Toolbox
      | Copyright MathWorks 2020
  u : Inport
  AND : Logic  IconShape=distinctive  AllPortsSameDT=off  OutDataTypeStr=boolean
  Compare To Zero : simulink/Logic and Bit Operations/Compare To Zero  relop=>  OutDataTypeStr=boolean
  Compare To Zero1 : simulink/Logic and Bit Operations/Compare To Zero  relop===  OutDataTypeStr=boolean
  Constant : Constant  Value=2*pi
  Constant1 : Constant  Value=pi
  Mod : Math  Operator=mod
  Mod1 : Math  Operator=mod
  Subtract : Sum
  Subtract1 : Sum  Inputs=+-
  Switch : Switch  Criteria=u2 > Threshold  SaturateOnIntegerOverflow=off  InputSameDT=off
  y : Outport
  wires:
  Subtract1/1 -> y/1
  Constant1/1 -> Subtract/2, Subtract1/2
  Mod1/1 -> Subtract1/1
  Constant/1 -> Mod1/2, Switch/1, Mod/2
  Subtract/1 -> Mod1/1
  Switch/1 -> Subtract/1
  Compare To Zero1/1 -> AND/2
  Mod/1 -> Switch/3
  u/1 -> Compare To Zero1/1, Compare To Zero/1, Mod/1
  Compare To Zero/1 -> AND/1
  AND/1 -> Switch/2

== stateflow chart FlutterSuppressionSystem/Test Assessment ==
  state step_1
  state step_2
    verify(dRatio > 0)
  (default) -> step_1
  step_1 -> step_2 : [
      | t >= 15
      | ]
  data: dRatio input

== matlab function FlutterSuppressionSystem/MATLAB Function ==
  settings: updateMethod=DISCRETE
  data: t input; dRatio output; pitch input
function dRatio = computeDampingRatio(t,pitch)
coder.extrinsic('exponentialFitAndPlot')
persistent Time;
persistent Data;
dRatio = 1;

% Append t and pitch to array
if isempty(Time)
    Time = t;
elseif t <= 15
    Time = [Time, t];
end

if isempty(Data)
    Data = pitch;
elseif t <= 15
    Data = [Data, pitch];
end

if t >= 15 || length(Data) > 15000
    % Find peaks
    % [~, peakIds] = findpeaks(Data,'minpeakheight', 0.002, 'minpeakdistance', 50);
    [~, peakIds] = findpeaks(Data, 'minpeakdistance', 50);
    
    if length(peakIds) >= 2
        peakTime= Time(peakIds);
        peakPos = Data(peakIds);
        rn = peakPos(1)./peakPos(2:end);
        L = 1:length(rn);
        
        % Find damping ratio
        dRatio = exponentialFitAndPlot(L, rn);
    else
        dRatio = 0.5;
    end

else
    dRatio = 0.5;
end

end

== stateflow chart FlutterSuppressionSystem/Test Sequence ==
  state step_1
    % Mach = [0.2, 0.4, 0.6, 1];
    % Altitude = [1000, 21000, 41000, 51000];
    Mach = Hecate_Mach;
    Altitude = Hecate_Alt;
  (default) -> step_1
  data: Mach output; Altitude output; Hecate_Mach parameter; Hecate_Alt parameter
